simulink model "mech_cambelt"  (Simulink 7.1)
settings: Solver=ode5  StartTime=0.0  StopTime=5  FixedStep=0.01  RelTol=1e-3
undefined symbols (not defined in the file or in its folder): m, rad, s, sigbuilder_block
libraries: mblibv1 x16
Description:
  | Cam Belt
  | 
  | Body rotates with a cam and a belt coupled to a pulley.
settings Model: Creator=jwendlan  LastModifiedBy=batserve  ExtModeAutoUpdateStatusClock=off
settings DataIOCC: SignalLoggingName=sigsOut  OutputOption=SpecifiedOutputTimes  OutputTimes=[0:0.1:10]
settings OptimizationCC: InlineInvariantSignals=on
settings DebuggingCC: SaveWithParameterizedLinksMsg=none  CheckExecutionContextPreStartOutputMsg=on  CheckExecutionContextRuntimeOutputMsg=on  SignalResolutionControl=TryResolveAllWithWarning  SolverPrmCheckMsg=none  MultiTaskDSMMsg=warning  MultiTaskCondExecSysMsg=none  SigSpecEnsureSampleTimeMsg=none  StrictBusMsg=None
settings HardwareCC: TargetBitPerLong=64  TargetEndianess=LittleEndian  TargetWordSize=64  TargetHWDeviceType=MATLAB Host  ProdEqTarget=off
settings RTWCC: SystemTargetFile=rsim.tlc  TemplateMakefile=rsim_default_tmf  Description=Rapid Simulation Target  ProcessScript=rsim_make_rtw_hook  IncludeERTFirstTime=on
settings RSimTargetCC: TargetFcnLib=ansi_tfl_tmw.mat  TargetFunctionLibrary=ANSI_C  IsPILTarget=off  EnableShiftOperators=on  PortableWordSizes=off
settings SimMechanicsCC: WarnOnRedundantConstraints=off  VisOnUpdateDiagram=on  VisDuringSimulation=on  VisConfigFile=mech_cambelt.mat

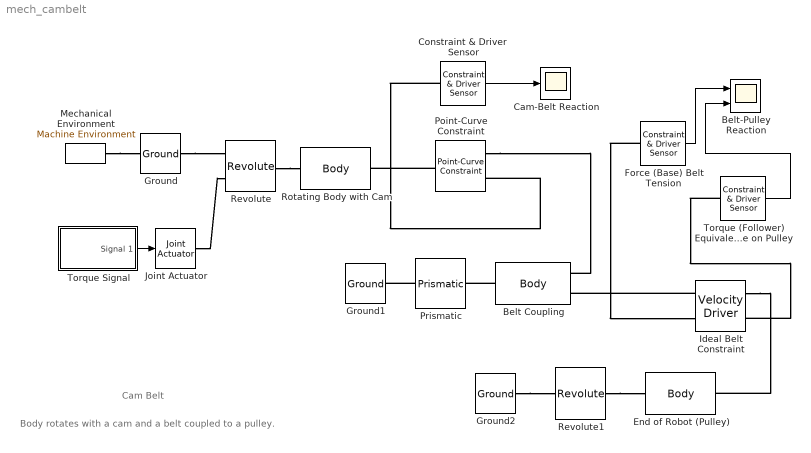
== system mech_cambelt ==
  note: Cam Belt
  note: Body rotates with a cam and
      | a belt coupled to a pulley.
  Belt Coupling : mblibv1/Bodies/Body  DialogController=MECH.DynMechDlgSource  PhysicalDomain=mechanical  SubClassName=Unknown  LeftPortType=workingframe  RightPortType=workingframe  LConnTagsString=CS1  RConnTagsString=CS2|CS3  DialogClass=MechanicalBodyBlock  Mass=1  MassUnits=kg  InertiaUnits=kg*m^2  Inertia=(2/5)*1*[0.02 0 0;0 1 0;0 0 1]  Shape=Cylinder  ShapeDims=[1 1]  ShapeUnits=m  ShapeUse=false  Density=1  DensityUnits=kg/m^3  DensityUse=false  GraphicsMode=1  BodyColor=[0.5 0.5 0.5]  GraphicsObj=[]  AttachedToCS=1  CG=Left$CG$[2 0 0]$WORLD$WORLD$m$[0 0 0]$Euler X-Y-Z$deg$WORLD$false  WorkingFrames=Left$CS1$[3 0 0]$WORLD$WORLD$m$[0 0 0]$Euler X-Y-Z$deg$WORLD$true#Right$CS2$[1 0 0]$WORLD$WORLD$m$[0 0 0]$Euler X-Y-Z$deg$WORLD$true#Right$CS3$[1 0 0]$WORLD$WORLD$m$[0 0 0]$Euler X-Y-Z$deg$WORLD$true  CGPos=[2 0 0]  CGRot=[0 0 0]  CS0Pos=[]  CS0Rot=[]  CS1Pos=[3 0 0]  CS1Rot=[0 0 0]  CS2Pos=[1 0 0]  CS2Rot=[0 0 0]  CS3Pos=[1 0 0]  CS3Rot=[0 0 0]  CS4Pos=[]  CS4Rot=[]  CS5Pos=[]  CS5Rot=[]  CS6Pos=[]  CS6Rot=[]  CS7Pos=[]  CS7Rot=[]  CS8Pos=[]  CS8Rot=[]  CS9Pos=[]  CS9Rot=[]  CS10Pos=[]  CS10Rot=[]  CS11Pos=[]  CS11Rot=[]  CS12Pos=[]  CS12Rot=[]  CS13Pos=[]  CS13Rot=[]  CS14Pos=[]  CS14Rot=[]  CS15Pos=[]  CS15Rot=[]  CS16Pos=[]  CS16Rot=[]  CS17Pos=[]  CS17Rot=[]  CS18Pos=[]  CS18Rot=[]  CS19Pos=[]  CS19Rot=[]  CS20Pos=[]  CS20Rot=[]
  Belt-Pulley Reaction : Scope  NumInputPorts=2
      settings: TimeRange=5  YMin=0~-25  YMax=25~0
  Cam-Belt Reaction : Scope
      settings: TimeRange=5  YMin=-50  YMax=10
  Constraint & Driver  Sensor : mblibv1/Sensors &  Actuators/Constraint & Driver  Sensor  DialogController=MECH.DynMechDlgSource  SystemSampleTime=-1  PhysicalDomain=Mechanical  DialogClass=ConstraintSensorBlock  SensedSide=Base  ReferenceFrame=Absolute (World)  ReactionForce=on  ForceUnits=N  ReactionMoment=on  MomentUnits=N-m  Muxed=on  OutputVector=[ 3 3 ]  ActiveIO=on  Width=6
  End of Robot (Pulley) : mblibv1/Bodies/Body  DialogController=MECH.DynMechDlgSource  PhysicalDomain=mechanical  SubClassName=Unknown  LeftPortType=workingframe  RightPortType=workingframe  LConnTagsString=CS1  RConnTagsString=CS2  DialogClass=MechanicalBodyBlock  Mass=1  MassUnits=kg  InertiaUnits=kg*m^2  Inertia=(2/5)*1*[0.5 0 0;0 0.5 0;0 0 1]  Shape=Cylinder  ShapeDims=[1 1]  ShapeUnits=m  ShapeUse=false  Density=1  DensityUnits=kg/m^3  DensityUse=false  GraphicsMode=1  BodyColor=[0.5 0.5 0.5]  GraphicsObj=[]  AttachedToCS=1  CG=Left$CG$[0 0 0]$CS1$CS1$m$[0 0 0]$Euler X-Y-Z$deg$WORLD$false  WorkingFrames=Left$CS1$[0 0 0]$ADJOINING$ADJOINING$m$[0 0 0]$Euler X-Y-Z$deg$WORLD$true#Right$CS2$[0 0 0]$CS1$CS1$m$[0 0 0]$Euler X-Y-Z$deg$WORLD$true#Right$CS3$[0 1 0]$CS1$CS1$m$[0 0 0]$Euler X-Y-Z$deg$WORLD$false#Right$CS4$[-1 0 0]$CS1$CS1$m$[0 0 0]$Euler X-Y-Z$deg$WORLD$false#Right$CS5$[0 -1 0]$CS1$CS1$m$[0 0 0]$Euler X-Y-Z$deg$WORLD$false#Right$CS6$[1 0 0]$CS1$CS1$m$[0 0 0]$Euler X-Y-Z$deg$WORLD$false  CGPos=[0 0 0]  CGRot=[0 0 0]  CS0Pos=[]  CS0Rot=[]  CS1Pos=[0 0 0]  CS1Rot=[0 0 0]  CS2Pos=[0 0 0]  CS2Rot=[0 0 0]  CS3Pos=[0 1 0]  CS3Rot=[0 0 0]  CS4Pos=[-1 0 0]  CS4Rot=[0 0 0]  CS5Pos=[0 -1 0]  CS5Rot=[0 0 0]  CS6Pos=[1 0 0]  CS6Rot=[0 0 0]  CS7Pos=[]  CS7Rot=[]  CS8Pos=[]  CS8Rot=[]  CS9Pos=[]  CS9Rot=[]  CS10Pos=[]  CS10Rot=[]  CS11Pos=[]  CS11Rot=[]  CS12Pos=[]  CS12Rot=[]  CS13Pos=[]  CS13Rot=[]  CS14Pos=[]  CS14Rot=[]  CS15Pos=[]  CS15Rot=[]  CS16Pos=[]  CS16Rot=[]  CS17Pos=[]  CS17Rot=[]  CS18Pos=[]  CS18Rot=[]  CS19Pos=[]  CS19Rot=[]  CS20Pos=[]  CS20Rot=[]
  Force (Base) Belt Tension : mblibv1/Sensors &  Actuators/Constraint & Driver  Sensor  DialogController=MECH.DynMechDlgSource  SystemSampleTime=-1  PhysicalDomain=Mechanical  DialogClass=ConstraintSensorBlock  SensedSide=Base  ReferenceFrame=Absolute (World)  ReactionForce=on  ForceUnits=N  ReactionMoment=off  MomentUnits=N-m  Muxed=on  OutputVector=[ 3 ]  ActiveIO=on  Width=3
  Ground : mblibv1/Bodies/Ground  DialogController=MECH.DynMechDlgSource  SystemSampleTime=-1  LeftPortType=env  RightPortType=workingframe  PhysicalDomain=Mechanical  DialogClass=GroundBlock  CoordPosition=[0 0 0]  CoordPositionUnits=m  StateVectorMgrId=-1  MachineId=[0 0]  ShowEnvPort=on
  Ground1 : mblibv1/Bodies/Ground  DialogController=MECH.DynMechDlgSource  SystemSampleTime=-1  LeftPortType=env  RightPortType=workingframe  PhysicalDomain=Mechanical  DialogClass=GroundBlock  CoordPosition=[3 0 0]  CoordPositionUnits=m  StateVectorMgrId=-1  MachineId=[0 0]  ShowEnvPort=off
  Ground2 : mblibv1/Bodies/Ground  DialogController=MECH.DynMechDlgSource  SystemSampleTime=-1  LeftPortType=env  RightPortType=workingframe  PhysicalDomain=Mechanical  DialogClass=GroundBlock  CoordPosition=[5 2 0]  CoordPositionUnits=m  StateVectorMgrId=-1  MachineId=[0 0]  ShowEnvPort=off
  Ideal Belt Constraint : mblibv1/Constraints &  Drivers/Velocity Driver  DialogController=MECH.DynMechDlgSource  PhysicalDomain=mechanical  SubClassName=Unknown  LeftPortType=blob  RightPortType=blob  LConnTagsString=__newl0|SA1  RConnTagsString=__newr0|SA1  DialogClass=ConstantVelocityConstraint  NumSAPorts=2  Unit_V=m/s  Unit_Omega=rad/s  Coef_V_Base=[1 0 0]  Csys_V_Base=WORLD  Coef_Omega_Base=[0 0 0]  Csys_Omega_Base=WORLD  Coef_V_Follower=[0 0 0]  Csys_V_Follower=WORLD  Coef_Omega_Follower=[0 0 1]  Csys_Omega_Follower=WORLD
  Joint Actuator : mblibv1/Sensors &  Actuators/Joint Actuator  DialogController=MECH.DynMechDlgSource  SystemSampleTime=-1  PhysicalDomain=Mechanical  PortType=blob  ActuationStyle=Force  AngleUnits=deg  ArcVelocityUnits=deg/s  ArcAccelerationUnits=deg/s^2  CoordPositionUnits=m  VelocityUnits=m/s  AccelerationUnits=m/s^2  ForceUnits=N  TorqueUnits=N-m  ActiveIO=on  Width=1  DialogClass=MechanicalActuatorBlock  Primitive=R1  ReferenceFrame=Absolute (INERTIAL)
  Mechanical Environment : mblibv1/Bodies/Machine Environment  Tag=Factory ground  DialogController=MECH.DialogSource  SystemSampleTime=-1  PortType=env  PhysicalDomain=Mechanical  DialogTemplateClass=MECH.MachineEnvironment  SyncWhenCopied=off  Gravity=[0 -9.81 0]  GravityUnits=m/s^2  GravityAsSignal=off  Dimensionality=3D Only  AnalysisType=Forward dynamics  LinearAssemblyTolerance=1e-3  LinearAssemblyToleranceUnits=m  AngularAssemblyTolerance=1e-3  AngularAssemblyToleranceUnits=rad  ConstraintSolverType=Stabilizing  ConstraintRelTolerance=1e-4  ConstraintAbsTolerance=1e-4  UseRobustSingularityHandling=off  RedundancyAnalysisToleranceType=Automatically select tolerance  RedundancyAnalysisTolerance=1e-14  StatePerturbationType=Fixed  PerturbationSize=1e-5  VisualizeMachine=on
  Point-Curve Constraint : mblibv1/Constraints &  Drivers/Point-Curve Constraint  Orientation=left  DialogController=MECH.DynMechDlgSource  PhysicalDomain=mechanical  SubClassName=Unknown  LeftPortType=blob  RightPortType=blob  LConnTagsString=__newl0|SA1  RConnTagsString=__newr0  DialogClass=PointCurveConstraint  Units=m  Xbreaks="[1     0.77547    0.058989    -0.52528    -0.55899    -0.17022     0.65485]"  Ybreaks="[0     0.42955     0.56832     0.29503    -0.12733    -0.36512    -0.39199]"  Zbreaks="[-0.0031056     0.36957     0.56832     0.29503    -0.12733    -0.46273    -0.40062]*0"  EndConditions=periodic  CanExtrapolate=off  NumSAPorts=1
  Prismatic : mblibv1/Joints/Prismatic  DialogController=MECH.DynMechDlgSource  PhysicalDomain=mechanical  SubClassName=Unknown  LeftPortType=blob  RightPortType=blob  LConnTagsString=__newl0  RConnTagsString=__newr0  NumSAPorts=0  CutJoint=off  MarkAsCut=off  Primitives=prismatic  PrimitiveProps=P1$WORLD$[-1 0 0]$prismatic  DialogClass=JointBlock  P1Axis=[-1 0 0]
  Revolute : mblibv1/Joints/Revolute  DialogController=MECH.DynMechDlgSource  PhysicalDomain=mechanical  SubClassName=Unknown  LeftPortType=blob  RightPortType=blob  LConnTagsString=__newl0|SA1  RConnTagsString=__newr0  NumSAPorts=1  CutJoint=off  MarkAsCut=off  Primitives=revolute  PrimitiveProps=R1$WORLD$[0 0 1]$revolute  DialogClass=JointBlock  R1Axis=[0 0 1]
  Revolute1 : mblibv1/Joints/Revolute  DialogController=MECH.DynMechDlgSource  PhysicalDomain=mechanical  SubClassName=Unknown  LeftPortType=blob  RightPortType=blob  LConnTagsString=__newl0  RConnTagsString=__newr0  NumSAPorts=0  CutJoint=off  MarkAsCut=off  Primitives=revolute  PrimitiveProps=R1$WORLD$[0 0 1]$revolute  DialogClass=JointBlock  R1Axis=[0 0 1]
  Rotating Body with Cam : mblibv1/Bodies/Body  DialogController=MECH.DynMechDlgSource  PhysicalDomain=mechanical  SubClassName=Unknown  LeftPortType=workingframe  RightPortType=workingframe  LConnTagsString=CS1  RConnTagsString=CS2  DialogClass=MechanicalBodyBlock  Mass=1  MassUnits=kg  InertiaUnits=kg*m^2  Inertia=(2/5)*1*[0.5 0 0;0 0.5 0;0 0 1]  Shape=Cylinder  ShapeDims=[1 1]  ShapeUnits=m  ShapeUse=false  Density=1  DensityUnits=kg/m^3  DensityUse=false  GraphicsMode=1  BodyColor=[0.5 0.5 0.5]  GraphicsObj=[]  AttachedToCS=1  CG=Left$CG$[0 0 0]$WORLD$WORLD$m$[0 0 0]$Euler X-Y-Z$deg$WORLD$false  WorkingFrames=Left$CS1$[0 0 0]$WORLD$WORLD$m$[0 0 0]$Euler X-Y-Z$deg$WORLD$true#Right$CS2$[0 0 0]$CS1$CS1$m$[0 0 0]$Euler X-Y-Z$deg$WORLD$true#Right$CS3$[0 1 0]$CS1$CS1$m$[0 0 0]$Euler X-Y-Z$deg$WORLD$false#Right$CS4$[-1 0 0]$CS1$CS1$m$[0 0 0]$Euler X-Y-Z$deg$WORLD$false#Right$CS5$[0 -1 0]$CS1$CS1$m$[0 0 0]$Euler X-Y-Z$deg$WORLD$false#Right$CS6$[1 0 0]$CS1$CS1$m$[0 0 0]$Euler X-Y-Z$deg$WORLD$false  CGPos=[0 0 0]  CGRot=[0 0 0]  CS0Pos=[]  CS0Rot=[]  CS1Pos=[0 0 0]  CS1Rot=[0 0 0]  CS2Pos=[0 0 0]  CS2Rot=[0 0 0]  CS3Pos=[0 1 0]  CS3Rot=[0 0 0]  CS4Pos=[-1 0 0]  CS4Rot=[0 0 0]  CS5Pos=[0 -1 0]  CS5Rot=[0 0 0]  CS6Pos=[1 0 0]  CS6Rot=[0 0 0]  CS7Pos=[]  CS7Rot=[]  CS8Pos=[]  CS8Rot=[]  CS9Pos=[]  CS9Rot=[]  CS10Pos=[]  CS10Rot=[]  CS11Pos=[]  CS11Rot=[]  CS12Pos=[]  CS12Rot=[]  CS13Pos=[]  CS13Rot=[]  CS14Pos=[]  CS14Rot=[]  CS15Pos=[]  CS15Rot=[]  CS16Pos=[]  CS16Rot=[]  CS17Pos=[]  CS17Rot=[]  CS18Pos=[]  CS18Rot=[]  CS19Pos=[]  CS19Rot=[]  CS20Pos=[]  CS20Rot=[]
  Torque Signal : Subsystem  Tag=STV Subsys  LoadFcn=sigbuilder_block('load');  StartFcn=sigbuilder_block('start');  StopFcn=sigbuilder_block('stop');  ClipboardFcn=sigbuilder_block('clipboard');  mask(Sigbuilder block){}
      mask help: Sigbuilder GUI
      mask init:
      | if ~strcmp(get_param(bdroot,'SimulationStatus'),'stopped') tuvar = sigbuilder_block('maskInit'); end
      settings: CopyFcn=sigbuilder_block('copy');  DeleteFcn=sigbuilder_block('delete');  ModelCloseFcn=sigbuilder_block('modelClose');  PreSaveFcn=sigbuilder_block('preSave');  NameChangeFcn=sigbuilder_block('namechange');  OpenFcn=sigbuilder_block('open',[57 48.75 519.75 399.75 ]);  CloseFcn=sigbuilder_block('close');
      mask Display: plot(0,0,100,100,[10,10,40,40,10],[80,20,20,80,80],[40,10],[50,50], [40,27,10],[65,72,56],[40,25,25,10],[28,28,43,43]);
  Torque (Follower) Equivalent Torque on Pulley : mblibv1/Sensors &  Actuators/Constraint & Driver  Sensor  DialogController=MECH.DynMechDlgSource  SystemSampleTime=-1  PhysicalDomain=Mechanical  DialogClass=ConstraintSensorBlock  SensedSide=Follower  ReferenceFrame=Absolute (World)  ReactionForce=off  ForceUnits=N  ReactionMoment=on  MomentUnits=N-m  Muxed=on  OutputVector=[ 3 ]  ActiveIO=on  Width=3
  wires:
  Torque Signal/1(Signal 1) -> Joint Actuator/1
  Constraint & Driver  Sensor/1 -> Cam-Belt Reaction/1
  Torque (Follower) Equivalent Torque on Pulley/1 -> Belt-Pulley Reaction/2
  Force (Base) Belt Tension/1 -> Belt-Pulley Reaction/1
  connections:
  Ground/RConn1 -- Revolute/LConn1
  Revolute/RConn1 -- Rotating Body with Cam/LConn1
  Joint Actuator/RConn1 -- Revolute/LConn2
  Prismatic/LConn1 -- Ground1/RConn1
  Belt Coupling/LConn1 -- Prismatic/RConn1
  Point-Curve Constraint/LConn1 -- Belt Coupling/RConn1
  Point-Curve Constraint/RConn1 -- Rotating Body with Cam/RConn1
  Constraint & Driver  Sensor/LConn1 -- Point-Curve Constraint/LConn2
  Ground2/RConn1 -- Revolute1/LConn1
  Revolute1/RConn1 -- End of Robot (Pulley)/LConn1
  Ideal Belt Constraint/RConn1 -- End of Robot (Pulley)/RConn1
  Ideal Belt Constraint/LConn1 -- Belt Coupling/RConn2
  Force (Base) Belt Tension/LConn1 -- Ideal Belt Constraint/LConn2
  Torque (Follower) Equivalent Torque on Pulley/LConn1 -- Ideal Belt Constraint/RConn2
  Mechanical Environment/RConn1 -- Ground/LConn1

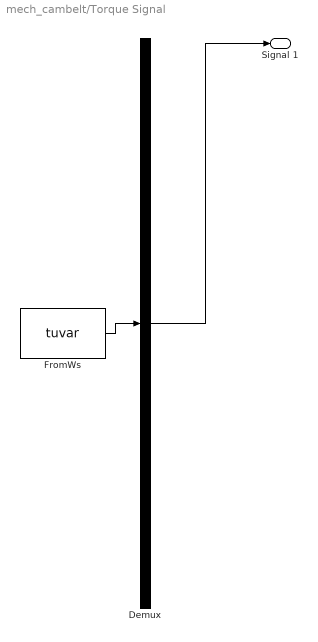
== system mech_cambelt/Torque Signal ==
  Demux : Demux  Tag=STV Demux  Outputs=1
  FromWs : FromWorkspace  Tag=STV FromWs  VariableName=tuvar  SampleTime=0  SigBuilderData=DataTag3  VnvData=DataTag4
      SigBuilderData=|
      | channels.label = 'Signal 1'
      | channels.allXData = {[0 0.58 0.58 1.16 1.94 1.94 10]}
      | channels.allYData = {[0 0 0.12 4.81 0.2 0.02 -0.12]}
      | dataSet.timeRange = [0 10]
      | dataSet.name = 'Group 1'
  Signal 1 : Outport  Tag=STV Outport  OutDataType=sfix(16)  OutScaling=2^0
  wires:
  Demux/1 -> Signal 1/1
  FromWs/1 -> Demux/1
